simulink model "TEST_simulink"  (R2022b)
settings: Solver=VariableStepAuto  StartTime=0.0  StopTime=10.0  RelTol=1e-3
undefined symbols (not defined in the file): c0, c1, GFl_Final_vlaue, GFl_Initial_value, GFl_P_primary, GFl_Q_set, GFl_Sample_time, GFl_Step_time, GFm_Final_vlaue, GFm_Initial_value, GFm_P_primary, GFm_Q_set, GFm_Sample_time, GFm_Step_time, GFm_V_set_phph, GFmAIC_f_set, GFmAIC_Final_vlaue, GFmAIC_Initial_value, GFmAIC_P_primary, GFmAIC_P_set, GFmAIC_Q_set, GFmAIC_Sample_time, GFmAIC_Step_time, l0, l1, r0, r1, SG_f_set, SG_Final_vlaue, SG_Initial_value, SG_P_primary, SG_Q_set, SG_Sample_time, SG_Step_time, SG_V_set_phph, sigbuilder_block, V1_L1, V1_Ph_Ph, V1_R1, V2_L1, V2_Ph_Ph, V2_R1
libraries: Model_DG_Grid_Forming_Converter x30, Model_DG_Grid_Following_Converter x15, simulink x15, Model_DG_Synchronous_Generator x15, spsThreePhaseVIMeasurementLib x14, spsThreePhasePISectionLineLib x14, spsThreePhaseBreakerLib x6, spsThreePhaseFaultLib x3, spsThreePhaseParallelRLCLoadLib x2, spsThreePhaseTransformerTwoWindingsLib x2, spspowerguiLib x1
(part 1 of 6)
settings Model: Creator=r.dong  LastModifiedBy=r.dong

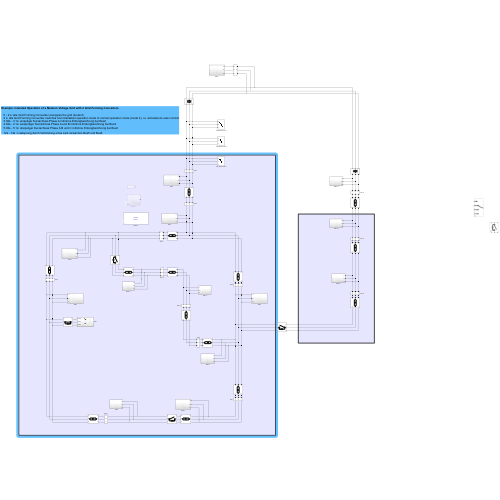
[thumbnail: Simulink's stored preview of the top-level diagram]
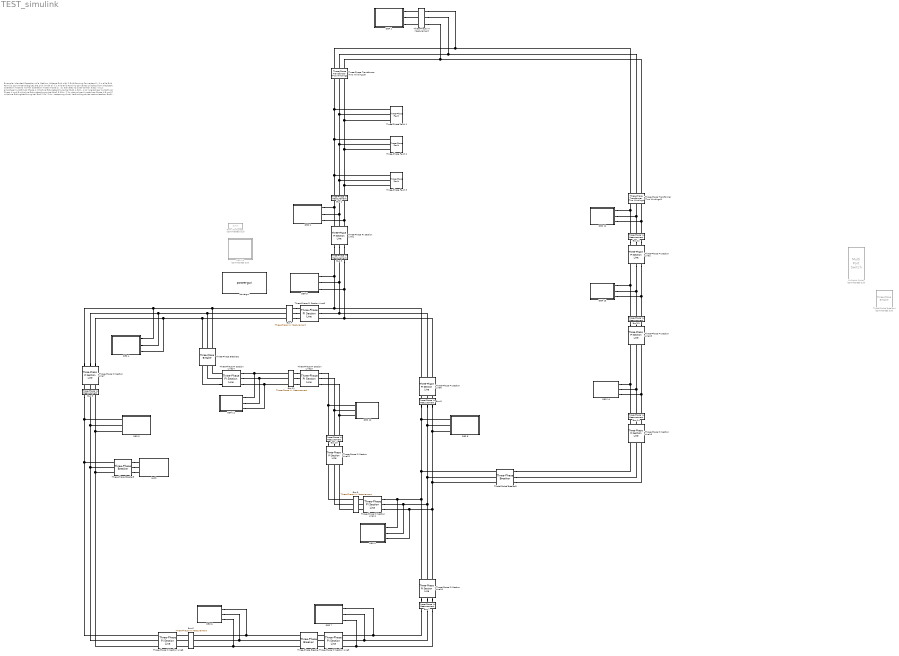
== system TEST_simulink ==
  note: Example: Islanded Operation of a Medium Voltage Grid with 2 Grid-Forming Converters
      |
      | 0 - 2 s: alle Grid Forming Conventer energizes the grid (mode 0)
      | 2 s: alle Grid Forming Conventer switches from blackstart operation mode to normal operation mode (mode 2), i.e. activates its outer control
      | 3.02s - 3.1s: einpoliger Kurzschluss Phase A mit/ohne Erdungberührung bei Bus2
      | 4.02s - 4.1s: zweipoliger Kurzschluss Phase A und B mit/ohne Erdungberührung bei Bus2
      | 5.02s - 5.1s: dreipoliger Kurzschluss Phase A B und C mit/ohne Erdungberührung bei Bus2
      |
      | 12s - 14s : Lastsprung durch Verbindung eines Last zwieschen Bus5 und Bus6
  Bus 10 : spsThreePhaseVIMeasurementLib/Three-Phase V-I Measurement  VoltageMeasurement=phase-to-phase  SetLabelV=on  LabelV=Vabc_10  Vpu=off  VpuLL=off  CurrentMeasurement=yes  SetLabelI=on  LabelI=Iabc_10  Ipu=off  Pbase=100e6  Vbase=500e3  OutputType=Complex  PhasorSimulation=off  PSBequivalent=0
  Bus 11 : spsThreePhaseVIMeasurementLib/Three-Phase V-I Measurement  VoltageMeasurement=phase-to-phase  SetLabelV=on  LabelV=Vabc_11  Vpu=off  VpuLL=off  CurrentMeasurement=yes  SetLabelI=on  LabelI=Iabc_11  Ipu=off  Pbase=100e6  Vbase=500e3  OutputType=Complex  PhasorSimulation=off  PSBequivalent=0
  Bus 12 : spsThreePhaseVIMeasurementLib/Three-Phase V-I Measurement  VoltageMeasurement=phase-to-phase  SetLabelV=on  LabelV=Vabc_12  Vpu=off  VpuLL=off  CurrentMeasurement=yes  SetLabelI=on  LabelI=Iabc_12  Ipu=off  Pbase=100e6  Vbase=500e3  OutputType=Complex  PhasorSimulation=off  PSBequivalent=0
  Bus 13 : spsThreePhaseVIMeasurementLib/Three-Phase V-I Measurement  VoltageMeasurement=phase-to-phase  SetLabelV=on  LabelV=Vabc_13  Vpu=off  VpuLL=off  CurrentMeasurement=yes  SetLabelI=on  LabelI=Iabc_13  Ipu=off  Pbase=100e6  Vbase=500e3  OutputType=Complex  PhasorSimulation=off  PSBequivalent=0
  Bus 14 : spsThreePhaseVIMeasurementLib/Three-Phase V-I Measurement  VoltageMeasurement=phase-to-phase  SetLabelV=on  LabelV=Vabc_14  Vpu=off  VpuLL=off  CurrentMeasurement=yes  SetLabelI=on  LabelI=Iabc_14  Ipu=off  Pbase=100e6  Vbase=500e3  OutputType=Complex  PhasorSimulation=off  PSBequivalent=0
  Bus 2 : spsThreePhaseVIMeasurementLib/Three-Phase V-I Measurement  VoltageMeasurement=phase-to-phase  SetLabelV=on  LabelV=Vabc_1  Vpu=off  VpuLL=off  CurrentMeasurement=yes  SetLabelI=on  LabelI=Iabc_1  Ipu=off  Pbase=100e6  Vbase=500e3  OutputType=Complex  PhasorSimulation=off  PSBequivalent=0
  Bus 3 : spsThreePhaseVIMeasurementLib/Three-Phase V-I Measurement  VoltageMeasurement=phase-to-ground  SetLabelV=on  LabelV=Vabc_3  Vpu=off  VpuLL=off  CurrentMeasurement=yes  SetLabelI=on  LabelI=Iabc_3  Ipu=off  Pbase=100e6  Vbase=500e3  OutputType=Complex  PhasorSimulation=off  PSBequivalent=0
  Bus 4 : spsThreePhaseVIMeasurementLib/Three-Phase V-I Measurement  VoltageMeasurement=phase-to-phase  SetLabelV=on  LabelV=Vabc_4  Vpu=off  VpuLL=off  CurrentMeasurement=yes  SetLabelI=on  LabelI=Iabc_4  Ipu=off  Pbase=100e6  Vbase=500e3  OutputType=Complex  PhasorSimulation=off  PSBequivalent=0
  Bus 5 : spsThreePhaseVIMeasurementLib/Three-Phase V-I Measurement  VoltageMeasurement=phase-to-phase  SetLabelV=on  LabelV=Vabc_5  Vpu=off  VpuLL=off  CurrentMeasurement=yes  SetLabelI=on  LabelI=Iabc_5  Ipu=off  Pbase=100e6  Vbase=500e3  OutputType=Complex  PhasorSimulation=off  PSBequivalent=0
  Bus 6 : spsThreePhaseVIMeasurementLib/Three-Phase V-I Measurement  VoltageMeasurement=phase-to-phase  SetLabelV=on  LabelV=Vabc_6  Vpu=off  VpuLL=off  CurrentMeasurement=yes  SetLabelI=on  LabelI=Iabc_6  Ipu=off  Pbase=100e6  Vbase=500e3  OutputType=Complex  PhasorSimulation=off  PSBequivalent=0
  Bus 7 : spsThreePhaseVIMeasurementLib/Three-Phase V-I Measurement  VoltageMeasurement=phase-to-phase  SetLabelV=on  LabelV=Vabc_7  Vpu=off  VpuLL=off  CurrentMeasurement=yes  SetLabelI=on  LabelI=Iabc_7  Ipu=off  Pbase=100e6  Vbase=500e3  OutputType=Complex  PhasorSimulation=off  PSBequivalent=0
  Bus 8 : spsThreePhaseVIMeasurementLib/Three-Phase V-I Measurement  VoltageMeasurement=phase-to-phase  SetLabelV=on  LabelV=Vabc_8  Vpu=off  VpuLL=off  CurrentMeasurement=yes  SetLabelI=on  LabelI=Iabc_8  Ipu=off  Pbase=100e6  Vbase=500e3  OutputType=Complex  PhasorSimulation=off  PSBequivalent=0
  Bus 9 : spsThreePhaseVIMeasurementLib/Three-Phase V-I Measurement  VoltageMeasurement=phase-to-phase  SetLabelV=on  LabelV=Vabc_9  Vpu=off  VpuLL=off  CurrentMeasurement=yes  SetLabelI=on  LabelI=Iabc_9  Ipu=off  Pbase=100e6  Vbase=500e3  OutputType=Complex  PhasorSimulation=off  PSBequivalent=0
  DER 1 : Subsystem
  DER 10 : Subsystem
  DER 11 : Subsystem
  DER 12 : Subsystem
  DER 13 : Subsystem
  DER 14 : Subsystem
  DER 15 : Subsystem  Commented=on
  DER 2 : Subsystem
  DER 3 : Subsystem
  DER 4 : Subsystem
  DER 5 : Subsystem
  DER 6 : Subsystem
  DER 7 : Subsystem
  DER 8 : Subsystem
  DER 9 : Subsystem
  From Workspace : FromWorkspace  Commented=on  VariableName=simin
  Last1 : Subsystem
  Multiport Switch : MultiPortSwitch  Commented=on  SaturateOnIntegerOverflow=off  InputSameDT=off
  Three-Phase PI Section Line1 : spsThreePhasePISectionLineLib/Three-Phase PI Section Line  LConnTagsString=a|b|c  RConnTagsString=A|B|C  Length=2.8  Frequency=50  Resistances=[ r1 r0]  Inductances="[ l1  l0]"  Capacitances=[c1 c0]
  Three-Phase PI Section Line10 : spsThreePhasePISectionLineLib/Three-Phase PI Section Line  LConnTagsString=a|b|c  RConnTagsString=A|B|C  Length=1.7  Frequency=50  Resistances=[ r1 r0]  Inductances="[ l1  l0]"  Capacitances=[c1 c0]
  Three-Phase PI Section Line11 : spsThreePhasePISectionLineLib/Three-Phase PI Section Line  LConnTagsString=a|b|c  RConnTagsString=A|B|C  Length=4.4  Frequency=50  Resistances=[ r1 r0]  Inductances="[ l1  l0]"  Capacitances=[c1 c0]
  Three-Phase PI Section Line12 : spsThreePhasePISectionLineLib/Three-Phase PI Section Line  LConnTagsString=a|b|c  RConnTagsString=A|B|C  Length=0.8  Frequency=50  Resistances=[ r1 r0]  Inductances="[ l1  l0]"  Capacitances=[c1 c0]
  Three-Phase PI Section Line13 : spsThreePhasePISectionLineLib/Three-Phase PI Section Line  LConnTagsString=a|b|c  RConnTagsString=A|B|C  Length=0.3  Frequency=50  Resistances=[ r1 r0]  Inductances="[ l1  l0]"  Capacitances=[c1 c0]
  Three-Phase PI Section Line14 : spsThreePhasePISectionLineLib/Three-Phase PI Section Line  LConnTagsString=a|b|c  RConnTagsString=A|B|C  Length=4.4  Frequency=50  Resistances=[ r1 r0]  Inductances="[ l1  l0]"  Capacitances=[c1 c0]
  Three-Phase PI Section Line15 : spsThreePhasePISectionLineLib/Three-Phase PI Section Line  LConnTagsString=a|b|c  RConnTagsString=A|B|C  Length=3  Frequency=50  Resistances=[ r1 r0]  Inductances="[ l1  l0]"  Capacitances=[c1 c0]
  Three-Phase PI Section Line16 : spsThreePhasePISectionLineLib/Three-Phase PI Section Line  LConnTagsString=a|b|c  RConnTagsString=A|B|C  Length=2  Frequency=50  Resistances=[ r1 r0]  Inductances="[ l1  l0]"  Capacitances=[c1 c0]
  Three-Phase PI Section Line2 : spsThreePhasePISectionLineLib/Three-Phase PI Section Line  LConnTagsString=a|b|c  RConnTagsString=A|B|C  Length=4.9  Frequency=50  Resistances=[ r1 r0]  Inductances="[ l1  l0]"  Capacitances=[c1 c0]
  Three-Phase PI Section Line5 : spsThreePhasePISectionLineLib/Three-Phase PI Section Line  LConnTagsString=a|b|c  RConnTagsString=A|B|C  Length=0.6  Frequency=50  Resistances=[ r1 r0]  Inductances="[ l1  l0]"  Capacitances=[c1 c0]
  Three-Phase PI Section Line6 : spsThreePhasePISectionLineLib/Three-Phase PI Section Line  LConnTagsString=a|b|c  RConnTagsString=A|B|C  Length=4.4  Frequency=50  Resistances=[ r1 r0]  Inductances="[ l1  l0]"  Capacitances=[c1 c0]
  Three-Phase PI Section Line7 : spsThreePhasePISectionLineLib/Three-Phase PI Section Line  LConnTagsString=a|b|c  RConnTagsString=A|B|C  Length=0.6  Frequency=50  Resistances=[ r1 r0]  Inductances="[ l1  l0]"  Capacitances=[c1 c0]
  Three-Phase PI Section Line8 : spsThreePhasePISectionLineLib/Three-Phase PI Section Line  LConnTagsString=a|b|c  RConnTagsString=A|B|C  Length=1.5  Frequency=50  Resistances=[ r1 r0]  Inductances="[ l1  l0]"  Capacitances=[c1 c0]
  Three-Phase PI Section Line9 : spsThreePhasePISectionLineLib/Three-Phase PI Section Line  LConnTagsString=a|b|c  RConnTagsString=A|B|C  Length=0.2  Frequency=50  Resistances=[ r1 r0]  Inductances="[ l1  l0]"  Capacitances=[c1 c0]
  Three-Phase Transformer (Two Windings)1 : spsThreePhaseTransformerTwoWindingsLib/Three-Phase Transformer (Two Windings)  Winding1Connection=Yg  Winding2Connection=Yg  CoreType=Three single-phase transformers  SetSaturation=off  Hysteresis=off  DataFile='hysteresis'  SetInitialFlux=off  Measurements=None  UNITS=pu  NominalPower=[ 1 , 50 ]  Winding1=[V1_Ph_Ph,V1_R1,V1_L1 ]  Winding2=[V2_Ph_Ph,V2_R1,V2_L1 ]  Rm=Rm  Lm=Lm  L0=0.5  Saturation=[ 0,0 ; 0.0024,1.2 ; 1.0,1.52 ]  InitialFluxes=[ 0.8 , -0.8 , 0.7 ]  BreakLoop=off  DiscreteSolver=Trapezoidal iterative  DataType=off  TransfoNumber=1
  Three-Phase Transformer (Two Windings)3 : spsThreePhaseTransformerTwoWindingsLib/Three-Phase Transformer (Two Windings)  Winding1Connection=Yg  Winding2Connection=Yg  CoreType=Three single-phase transformers  SetSaturation=off  Hysteresis=off  DataFile='hysteresis'  SetInitialFlux=off  Measurements=None  UNITS=pu  NominalPower=[ 1 , 50 ]  Winding1=[V1_Ph_Ph,V1_R1,V1_L1 ]  Winding2=[V2_Ph_Ph,V2_R1,V2_L1 ]  Rm=Rm  Lm=Lm  L0=0.5  Saturation=[ 0,0 ; 0.0024,1.2 ; 1.0,1.52 ]  InitialFluxes=[ 0.8 , -0.8 , 0.7 ]  BreakLoop=off  DiscreteSolver=Trapezoidal iterative  DataType=off  TransfoNumber=1
  Three-Phase V-I Measurement : spsThreePhaseVIMeasurementLib/Three-Phase V-I Measurement  VoltageMeasurement=no  SetLabelV=off  LabelV=Vabc  Vpu=off  VpuLL=off  CurrentMeasurement=no  SetLabelI=off  LabelI=Iabc  Ipu=off  Pbase=100e6  Vbase=500e3  OutputType=Complex  PhasorSimulation=off  PSBequivalent=0
  Three-Phase Breaker1 : spsThreePhaseBreakerLib/Three-Phase Breaker  InitialState=open  SwitchA=on  SwitchB=on  SwitchC=on  SwitchTimes=Break1_switching_time  External=off  BreakerResistance=Break1_Ron  SnubberResistance=Break1_Rs  SnubberCapacitance=Break1_Cs  Measurements=None
  Three-Phase Breaker2 : spsThreePhaseBreakerLib/Three-Phase Breaker  InitialState=open  SwitchA=on  SwitchB=on  SwitchC=on  SwitchTimes=Break2_switching_time  External=off  BreakerResistance=Break2_Ron  SnubberResistance=Break2_Rs  SnubberCapacitance=Break2_Cs  Measurements=None
  Three-Phase Breaker3 : spsThreePhaseBreakerLib/Three-Phase Breaker  InitialState=open  SwitchA=on  SwitchB=on  SwitchC=on  SwitchTimes=Break3_switching_time  External=off  BreakerResistance=Break3_Ron  SnubberResistance=Break3_Rs  SnubberCapacitance=Break3_Cs  Measurements=None
  Three-Phase Breaker4 : spsThreePhaseBreakerLib/Three-Phase Breaker  Commented=on  InitialState=open  SwitchA=on  SwitchB=on  SwitchC=on  SwitchTimes=Break2_switching_time  External=off  BreakerResistance=Break2_Ron  SnubberResistance=Break2_Rs  SnubberCapacitance=Break2_Cs  Measurements=None
  Three-Phase Breaker5 : spsThreePhaseBreakerLib/Three-Phase Breaker  InitialState=closed  SwitchA=on  SwitchB=on  SwitchC=on  SwitchTimes=14  External=off  BreakerResistance=Break2_Ron  SnubberResistance=Break2_Rs  SnubberCapacitance=Break2_Cs  Measurements=None
  Three-Phase Fault 1 : spsThreePhaseFaultLib/Three-Phase Fault  InitialStates=0  FaultA=on  FaultB=off  FaultC=off  GroundFault=off  SwitchTimes=Fault1_Break_switching_time  External=off  SwitchStatus=NaN  FaultResistance=Fault1_Ron  GroundResistance=Fault1_Rg  SnubberResistance=Fault1_Rs  SnubberCapacitance=Fault1_Cs  Measurements=None
  Three-Phase Fault 2 : spsThreePhaseFaultLib/Three-Phase Fault  InitialStates=0  FaultA=on  FaultB=on  FaultC=off  GroundFault=off  SwitchTimes=Fault2_Break_switching_time  External=off  SwitchStatus=NaN  FaultResistance=Fault2_Ron  GroundResistance=Fault2_Rg  SnubberResistance=Fault2_Rs  SnubberCapacitance=Fault2_Cs  Measurements=None
  Three-Phase Fault 3 : spsThreePhaseFaultLib/Three-Phase Fault  InitialStates=0  FaultA=on  FaultB=on  FaultC=on  GroundFault=off  SwitchTimes=Fault3_Break_switching_time  External=off  SwitchStatus=NaN  FaultResistance=Fault3_Ron  GroundResistance=Fault3_Rg  SnubberResistance=Fault3_Rs  SnubberCapacitance=Fault3_Cs  Measurements=None
  powergui : spspowerguiLib/powergui  Priority=1  SimulationMode=Discrete  SampleTime=1e-4  frequency=60  Iterations=50  frequencyindice=0  Pbase=100e6  ErrMax=1e-4  UnitsV=kV  UnitsW=MW  buscounter=0  FunctionMessages=off  echomessages=off  EnableUseOfTLC=off  CurrentSourceSwitches=off  DisableSnubberDevices=off  DisableRonSwitches=off  DisableVfSwitches=off  DisplayEquations=off  AutomaticDiscreteSolvers=off  SolverType=Backward Euler  Interpol=off  ExternalGateDelay=off  methode=off  Ts=100  x0status=blocks  SPID=on  SwTol=0  HookPort=off  NonlinearTolerance=1e-4  nMaxIteration=100  ContinueOnMaxIteration=off  RestoreLinks=warning  ResistiveCurrentMeasurement=off  Frange=[0:2:500]  Ylog=off  Xlog=on  ShowGrid=off  save=off  variable=ZData  structure=0  ZoomFFT=off  StartTime=0.0  cycles=1  DisplayStyle=1  fundamental=60  FreqAxis=off  MaxFrequency=1000  frequencyindicesteady=1  RmsSteady=1  display=off
  connections:
  Three-Phase PI Section Line5/LConn1 -- Three-Phase PI Section Line6/LConn1 -- DER 3/RConn1 -- Bus 3/RConn1
  Bus 12/LConn2 -- DER 12/RConn2 -- Three-Phase Transformer (Two Windings)1/RConn2
  Three-Phase Breaker3/LConn1 -- Three-Phase PI Section Line16/RConn1
  Three-Phase Breaker1/LConn3 -- Bus 6/RConn3 -- DER 6/RConn3
  Three-Phase Breaker1/LConn1 -- Bus 6/RConn1 -- DER 6/RConn1
  Bus 12/LConn3 -- DER 12/RConn3 -- Three-Phase Transformer (Two Windings)1/RConn3
  Three-Phase PI Section Line13/LConn1 -- Bus 10/RConn1 -- DER 10/RConn1
  Three-Phase PI Section Line6/LConn2 -- Three-Phase PI Section Line5/LConn2 -- DER 3/RConn2 -- Bus 3/RConn2
  Three-Phase PI Section Line8/LConn3 -- Bus 5/RConn3 -- DER 5/RConn3 -- Three-Phase Breaker5/LConn3
  Bus 5/RConn2 -- DER 5/RConn2 -- Three-Phase Breaker5/LConn2 -- Three-Phase PI Section Line8/LConn2
  Bus 9/LConn3 -- Three-Phase PI Section Line12/LConn3
  Three-Phase PI Section Line2/RConn3 -- DER 13/RConn3 -- Bus 13/LConn3
  Three-Phase PI Section Line13/LConn3 -- DER 10/RConn3 -- Bus 10/RConn3
  Three-Phase PI Section Line14/LConn3 -- Bus 11/RConn3 -- DER 11/RConn3
  Three-Phase PI Section Line11/LConn2 -- Bus 8/LConn2 -- DER 8/RConn2 -- Three-Phase Breaker3/RConn2 -- Three-Phase PI Section Line10/RConn2 -- DER 9/RConn2
  Bus 5/RConn1 -- DER 5/RConn1 -- Three-Phase Breaker5/LConn1 -- Three-Phase PI Section Line8/LConn1
  Bus 9/LConn2 -- Three-Phase PI Section Line12/LConn2
  Three-Phase Transformer (Two Windings)1/LConn1 -- Three-Phase V-I Measurement/RConn1 -- Three-Phase Transformer (Two Windings)3/LConn1
  Three-Phase PI Section Line7/LConn1 -- Three-Phase Breaker2/LConn1 -- Bus 4/RConn1 -- DER 4/RConn1
  Three-Phase PI Section Line2/RConn2 -- DER 13/RConn2 -- Bus 13/LConn2
  Three-Phase PI Section Line11/LConn3 -- DER 8/RConn3 -- Bus 8/LConn3 -- Three-Phase Breaker3/RConn3 -- Three-Phase PI Section Line10/RConn3 -- DER 9/RConn3
  Bus 9/LConn1 -- Three-Phase PI Section Line12/LConn1
  Three-Phase Breaker3/LConn2 -- Three-Phase PI Section Line16/RConn2
  Three-Phase Breaker3/RConn1 -- Bus 8/LConn1 -- DER 8/RConn1 -- DER 9/RConn1 -- Three-Phase PI Section Line11/LConn1 -- Three-Phase PI Section Line10/RConn1
  Three-Phase PI Section Line13/LConn2 -- Bus 10/RConn2 -- DER 10/RConn2
  Three-Phase Breaker1/LConn2 -- Bus 6/RConn2 -- DER 6/RConn2
  Three-Phase Transformer (Two Windings)3/LConn2 -- Three-Phase V-I Measurement/RConn2 -- Three-Phase Transformer (Two Windings)1/LConn2
  Three-Phase Breaker2/LConn2 -- DER 4/RConn2 -- Three-Phase PI Section Line7/LConn2 -- Bus 4/RConn2
  Bus 7/LConn1 -- DER 7/RConn1 -- Three-Phase PI Section Line9/RConn1
  Bus 13/LConn1 -- DER 13/RConn1 -- Three-Phase PI Section Line2/RConn1
  Bus 7/LConn2 -- Three-Phase PI Section Line9/RConn2 -- DER 7/RConn2
  Three-Phase PI Section Line7/LConn3 -- Three-Phase Breaker2/LConn3 -- Bus 4/RConn3 -- DER 4/RConn3
  Three-Phase PI Section Line1/LConn3 -- DER 2/RConn3 -- Bus 2/RConn3
  Three-Phase PI Section Line5/LConn3 -- Three-Phase PI Section Line6/LConn3 -- DER 3/RConn3 -- Bus 3/RConn3
  Bus 12/LConn1 -- DER 12/RConn1 -- Three-Phase Transformer (Two Windings)1/RConn1
  Three-Phase PI Section Line1/LConn1 -- DER 2/RConn1 -- Bus 2/RConn1
  Three-Phase PI Section Line14/LConn2 -- DER 11/RConn2 -- Bus 11/RConn2
  Three-Phase Breaker3/LConn3 -- Three-Phase PI Section Line16/RConn3
  Bus 7/LConn3 -- Three-Phase PI Section Line9/RConn3 -- DER 7/RConn3
  Three-Phase Transformer (Two Windings)1/LConn3 -- Three-Phase V-I Measurement/RConn3 -- Three-Phase Transformer (Two Windings)3/LConn3
  Three-Phase PI Section Line1/LConn2 -- DER 2/RConn2 -- Bus 2/RConn2
  Bus 13/RConn2 -- Three-Phase PI Section Line15/LConn2
  Bus 4/LConn2 -- Three-Phase PI Section Line5/RConn2
  Bus 13/RConn3 -- Three-Phase PI Section Line15/LConn3
  Three-Phase PI Section Line10/LConn3 -- Bus 7/RConn3
  Bus 12/RConn1 -- Three-Phase PI Section Line2/LConn1
  Bus 12/RConn3 -- Three-Phase PI Section Line2/LConn3
  Bus 6/LConn2 -- Three-Phase PI Section Line8/RConn2
  Bus 5/LConn2 -- Three-Phase PI Section Line7/RConn2
  Bus 14/LConn2 -- DER 14/RConn2 -- Three-Phase PI Section Line15/RConn2
  Three-Phase Fault 1/LConn3 -- Three-Phase Transformer (Two Windings)3/RConn3 -- Three-Phase Fault 3/LConn3 -- Bus 2/LConn3 -- Three-Phase Fault 2/LConn3
  Three-Phase PI Section Line1/RConn3 -- Bus 3/LConn3
  Three-Phase Fault 1/LConn2 -- Three-Phase Transformer (Two Windings)3/RConn2 -- Three-Phase Fault 2/LConn2 -- Three-Phase Fault 3/LConn2 -- Bus 2/LConn2
  Bus 13/RConn1 -- Three-Phase PI Section Line15/LConn1
  Three-Phase PI Section Line16/LConn1 -- Bus 14/RConn1
  Bus 10/LConn2 -- Three-Phase PI Section Line12/RConn2
  Three-Phase PI Section Line11/RConn1 -- Bus 9/RConn1
  Three-Phase PI Section Line16/LConn3 -- Bus 14/RConn3
  Bus 4/LConn3 -- Three-Phase PI Section Line5/RConn3
  Bus 10/LConn1 -- Three-Phase PI Section Line12/RConn1
  Three-Phase Fault 1/LConn1 -- Three-Phase Transformer (Two Windings)3/RConn1 -- Three-Phase Fault 2/LConn1 -- Three-Phase Fault 3/LConn1 -- Bus 2/LConn1
  Bus 14/LConn1 -- DER 14/RConn1 -- Three-Phase PI Section Line15/RConn1
  Bus 5/LConn3 -- Three-Phase PI Section Line7/RConn3
  Bus 10/LConn3 -- Three-Phase PI Section Line12/RConn3
  Bus 11/LConn3 -- Three-Phase PI Section Line13/RConn3
  Three-Phase PI Section Line11/RConn2 -- Bus 9/RConn2
  Three-Phase PI Section Line14/RConn1 -- Three-Phase Breaker2/RConn1
  Three-Phase PI Section Line16/LConn2 -- Bus 14/RConn2
  Bus 6/LConn3 -- Three-Phase PI Section Line8/RConn3
  Three-Phase PI Section Line6/RConn3 -- Bus 8/RConn3
  Three-Phase PI Section Line6/RConn2 -- Bus 8/RConn2
  Three-Phase PI Section Line14/RConn2 -- Three-Phase Breaker2/RConn2
  Three-Phase PI Section Line9/LConn1 -- Three-Phase Breaker1/RConn1
  Bus 11/LConn2 -- Three-Phase PI Section Line13/RConn2
  Three-Phase PI Section Line10/LConn1 -- Bus 7/RConn1
  Three-Phase PI Section Line14/RConn3 -- Three-Phase Breaker2/RConn3
  Three-Phase PI Section Line1/RConn1 -- Bus 3/LConn1
  Bus 6/LConn1 -- Three-Phase PI Section Line8/RConn1
  Three-Phase PI Section Line6/RConn1 -- Bus 8/RConn1
  Three-Phase PI Section Line11/RConn3 -- Bus 9/RConn3
  Bus 11/LConn1 -- Three-Phase PI Section Line13/RConn1
  Three-Phase PI Section Line9/LConn3 -- Three-Phase Breaker1/RConn3
  Three-Phase PI Section Line10/LConn2 -- Bus 7/RConn2
  Three-Phase PI Section Line9/LConn2 -- Three-Phase Breaker1/RConn2
  Bus 4/LConn1 -- Three-Phase PI Section Line5/RConn1
  Bus 12/RConn2 -- Three-Phase PI Section Line2/LConn2
  Three-Phase PI Section Line1/RConn2 -- Bus 3/LConn2
  Bus 5/LConn1 -- Three-Phase PI Section Line7/RConn1
  Bus 14/LConn3 -- DER 14/RConn3 -- Three-Phase PI Section Line15/RConn3
  Three-Phase PI Section Line14/LConn1 -- DER 11/RConn1 -- Bus 11/RConn1
  DER 1/RConn1 -- Three-Phase V-I Measurement/LConn1
  DER 1/RConn2 -- Three-Phase V-I Measurement/LConn2
  DER 1/RConn3 -- Three-Phase V-I Measurement/LConn3
  Three-Phase Breaker5/RConn1 -- Last1/LConn1
  Three-Phase Breaker5/RConn2 -- Last1/LConn2
  Three-Phase Breaker5/RConn3 -- Last1/LConn3

== system TEST_simulink/DER 1 ==
  Grid Following Conventer : Subsystem  Commented=on
  Grid Forming Conventer : Subsystem  Commented=on
  Grid Forming Converter AIC : Subsystem  Commented=on
  SG : Subsystem
  L1 : PMIOPort  Side=Right
  L2 : PMIOPort  Port=2  Side=Right
  L3 : PMIOPort  Port=3  Side=Right
  connections:
  SG/RConn1 -- Grid Forming Converter AIC/RConn1 -- L1/RConn1 -- Grid Forming Converter AIC/RConn3 -- Grid Forming Converter AIC/RConn2 -- Grid Forming Conventer/RConn1 -- Grid Following Conventer/RConn1
  SG/RConn2 -- L2/RConn1 -- Grid Forming Conventer/RConn2 -- Grid Following Conventer/RConn2
  SG/RConn3 -- L3/RConn1 -- Grid Forming Conventer/RConn3 -- Grid Following Conventer/RConn3

== system TEST_simulink/DER 10 ==
  Grid Following Conventer : Subsystem  Commented=on
  Grid Forming Conventer : Subsystem  Commented=on
  Grid Forming Converter AIC : Subsystem  Commented=on
  SG : Subsystem  Commented=on
  L1 : PMIOPort  Side=Right
  L2 : PMIOPort  Port=2  Side=Right
  L3 : PMIOPort  Port=3  Side=Right
  connections:
  L3/RConn1 -- SG/RConn3 -- Grid Following Conventer/RConn3 -- Grid Forming Conventer/RConn3
  L2/RConn1 -- SG/RConn2 -- Grid Following Conventer/RConn2 -- Grid Forming Conventer/RConn2
  L1/RConn1 -- Grid Forming Converter AIC/RConn1 -- SG/RConn1 -- Grid Following Conventer/RConn1 -- Grid Forming Conventer/RConn1 -- Grid Forming Converter AIC/RConn2 -- Grid Forming Converter AIC/RConn3

== system TEST_simulink/DER 11 ==
  Grid Following Conventer : Subsystem  Commented=on
  Grid Forming Conventer : Subsystem  Commented=on
  Grid Forming Converter AIC : Subsystem  Commented=on
  SG : Subsystem  Commented=on
  L1 : PMIOPort  Side=Right
  L2 : PMIOPort  Port=2  Side=Right
  L3 : PMIOPort  Port=3  Side=Right
  connections:
  Grid Forming Converter AIC/RConn3 -- Grid Forming Converter AIC/RConn2 -- Grid Forming Conventer/RConn1 -- Grid Following Conventer/RConn1 -- SG/RConn1 -- Grid Forming Converter AIC/RConn1 -- L1/RConn1
  Grid Forming Conventer/RConn2 -- Grid Following Conventer/RConn2 -- SG/RConn2 -- L2/RConn1
  Grid Forming Conventer/RConn3 -- Grid Following Conventer/RConn3 -- SG/RConn3 -- L3/RConn1

== system TEST_simulink/DER 12 ==
  Grid Following Conventer : Subsystem  Commented=on
  Grid Forming Conventer : Subsystem  Commented=on
  Grid Forming Converter AIC : Subsystem  Commented=on
  SG : Subsystem  Commented=on
  L1 : PMIOPort  Side=Right
  L2 : PMIOPort  Port=2  Side=Right
  L3 : PMIOPort  Port=3  Side=Right
  connections:
  Grid Forming Converter AIC/RConn3 -- Grid Forming Converter AIC/RConn2 -- Grid Forming Conventer/RConn1 -- Grid Following Conventer/RConn1 -- SG/RConn1 -- Grid Forming Converter AIC/RConn1 -- L1/RConn1
  Grid Forming Conventer/RConn2 -- Grid Following Conventer/RConn2 -- SG/RConn2 -- L2/RConn1
  Grid Forming Conventer/RConn3 -- Grid Following Conventer/RConn3 -- SG/RConn3 -- L3/RConn1

== system TEST_simulink/DER 13 ==
  Grid Following Conventer : Subsystem  Commented=on
  Grid Forming Conventer : Subsystem  Commented=on
  Grid Forming Converter AIC : Subsystem  Commented=on
  SG : Subsystem  Commented=on
  L1 : PMIOPort  Side=Right
  L2 : PMIOPort  Port=2  Side=Right
  L3 : PMIOPort  Port=3  Side=Right
  connections:
  Grid Forming Converter AIC/RConn3 -- Grid Forming Converter AIC/RConn2 -- Grid Forming Conventer/RConn1 -- Grid Following Conventer/RConn1 -- SG/RConn1 -- Grid Forming Converter AIC/RConn1 -- L1/RConn1
  Grid Forming Conventer/RConn2 -- Grid Following Conventer/RConn2 -- SG/RConn2 -- L2/RConn1
  Grid Forming Conventer/RConn3 -- Grid Following Conventer/RConn3 -- SG/RConn3 -- L3/RConn1

== system TEST_simulink/DER 14 ==
  Grid Following Conventer : Subsystem  Commented=on
  Grid Forming Conventer : Subsystem  Commented=on
  Grid Forming Converter AIC : Subsystem  Commented=on
  SG : Subsystem  Commented=on
  L1 : PMIOPort  Side=Right
  L2 : PMIOPort  Port=2  Side=Right
  L3 : PMIOPort  Port=3  Side=Right
  connections:
  Grid Forming Converter AIC/RConn3 -- Grid Forming Converter AIC/RConn2 -- Grid Forming Conventer/RConn1 -- Grid Following Conventer/RConn1 -- SG/RConn1 -- Grid Forming Converter AIC/RConn1 -- L1/RConn1
  Grid Forming Conventer/RConn2 -- Grid Following Conventer/RConn2 -- SG/RConn2 -- L2/RConn1
  Grid Forming Conventer/RConn3 -- Grid Following Conventer/RConn3 -- SG/RConn3 -- L3/RConn1

== system TEST_simulink/DER 15 ==
  Grid Following Conventer : Subsystem  Commented=on
  Grid Forming Conventer : Subsystem  Commented=on
  Grid Forming Converter AIC : Subsystem  Commented=on
  SG : Subsystem  Commented=on
  L1 : PMIOPort  Side=Right
  L2 : PMIOPort  Port=2  Side=Right
  L3 : PMIOPort  Port=3  Side=Right
  connections:
  L3/RConn1 -- SG/RConn3 -- Grid Following Conventer/RConn3 -- Grid Forming Conventer/RConn3
  L2/RConn1 -- SG/RConn2 -- Grid Following Conventer/RConn2 -- Grid Forming Conventer/RConn2
  L1/RConn1 -- Grid Forming Converter AIC/RConn1 -- SG/RConn1 -- Grid Following Conventer/RConn1 -- Grid Forming Conventer/RConn1 -- Grid Forming Converter AIC/RConn2 -- Grid Forming Converter AIC/RConn3

== system TEST_simulink/DER 2 ==
  Grid Following Conventer : Subsystem  Commented=on
  Grid Forming Conventer : Subsystem  Commented=on
  Grid Forming Converter AIC : Subsystem  Commented=on
  SG : Subsystem  Commented=on
  L1 : PMIOPort  Side=Right
  L2 : PMIOPort  Port=2  Side=Right
  L3 : PMIOPort  Port=3  Side=Right
  connections:
  L3/RConn1 -- SG/RConn3 -- Grid Following Conventer/RConn3 -- Grid Forming Conventer/RConn3
  L2/RConn1 -- SG/RConn2 -- Grid Following Conventer/RConn2 -- Grid Forming Conventer/RConn2
  L1/RConn1 -- Grid Forming Converter AIC/RConn1 -- SG/RConn1 -- Grid Following Conventer/RConn1 -- Grid Forming Conventer/RConn1 -- Grid Forming Converter AIC/RConn2 -- Grid Forming Converter AIC/RConn3

== system TEST_simulink/DER 3 ==
  Grid Following Conventer : Subsystem  Commented=on
  Grid Forming Conventer : Subsystem  Commented=on
  Grid Forming Converter AIC : Subsystem  Commented=on
  SG : Subsystem  Commented=on
  L1 : PMIOPort  Side=Right
  L2 : PMIOPort  Port=2  Side=Right
  L3 : PMIOPort  Port=3  Side=Right
  connections:
  Grid Forming Converter AIC/RConn2 -- Grid Forming Converter AIC/RConn1 -- Grid Forming Conventer/RConn1 -- Grid Following Conventer/RConn1 -- SG/RConn1 -- Grid Forming Converter AIC/RConn3 -- L1/RConn1
  Grid Following Conventer/RConn2 -- SG/RConn2 -- Grid Forming Conventer/RConn2 -- L2/RConn1
  Grid Following Conventer/RConn3 -- SG/RConn3 -- Grid Forming Conventer/RConn3 -- L3/RConn1

== system TEST_simulink/DER 4 ==
  Grid Following Conventer : Subsystem  Commented=on
  Grid Forming Conventer : Subsystem  Commented=on
  Grid Forming Converter AIC : Subsystem  Commented=on
  SG : Subsystem  Commented=on
  L1 : PMIOPort  Side=Right
  L2 : PMIOPort  Port=2  Side=Right
  L3 : PMIOPort  Port=3  Side=Right
  connections:
  L3/RConn1 -- Grid Forming Conventer/RConn3 -- SG/RConn3 -- Grid Following Conventer/RConn3
  L2/RConn1 -- Grid Forming Conventer/RConn2 -- SG/RConn2 -- Grid Following Conventer/RConn2
  L1/RConn1 -- Grid Forming Converter AIC/RConn3 -- Grid Forming Converter AIC/RConn2 -- Grid Forming Converter AIC/RConn1 -- Grid Forming Conventer/RConn1 -- SG/RConn1 -- Grid Following Conventer/RConn1

== system TEST_simulink/DER 5 ==
  Grid Following Conventer : Subsystem  Commented=on
  Grid Forming Conventer : Subsystem  Commented=on
  Grid Forming Converter AIC : Subsystem  Commented=on
  SG : Subsystem  Commented=on
  L1 : PMIOPort  Side=Right
  L2 : PMIOPort  Port=2  Side=Right
  L3 : PMIOPort  Port=3  Side=Right
  connections:
  L3/RConn1 -- Grid Forming Conventer/RConn3 -- SG/RConn3 -- Grid Following Conventer/RConn3
  Grid Following Conventer/RConn2 -- SG/RConn2 -- Grid Forming Conventer/RConn2 -- L2/RConn1
  L1/RConn1 -- Grid Forming Converter AIC/RConn3 -- Grid Forming Converter AIC/RConn2 -- Grid Forming Converter AIC/RConn1 -- Grid Forming Conventer/RConn1 -- SG/RConn1 -- Grid Following Conventer/RConn1

== system TEST_simulink/DER 6 ==
  Grid Following Conventer : Subsystem  Commented=on
  Grid Forming Conventer : Subsystem  Commented=on
  Grid Forming Converter AIC : Subsystem  Commented=on
  SG : Subsystem  Commented=on
  L1 : PMIOPort  Side=Right
  L2 : PMIOPort  Port=2  Side=Right
  L3 : PMIOPort  Port=3  Side=Right
  connections:
  Grid Forming Converter AIC/RConn3 -- Grid Forming Converter AIC/RConn2 -- Grid Forming Conventer/RConn1 -- Grid Following Conventer/RConn1 -- SG/RConn1 -- Grid Forming Converter AIC/RConn1 -- L1/RConn1
  Grid Forming Conventer/RConn2 -- Grid Following Conventer/RConn2 -- SG/RConn2 -- L2/RConn1
  Grid Forming Conventer/RConn3 -- Grid Following Conventer/RConn3 -- SG/RConn3 -- L3/RConn1

== system TEST_simulink/DER 7 ==
  Grid Following Conventer : Subsystem  Commented=on
  Grid Forming Conventer : Subsystem  Commented=on
  Grid Forming Converter AIC : Subsystem  Commented=on
  SG : Subsystem  Commented=on
  L1 : PMIOPort  Side=Right
  L2 : PMIOPort  Port=2  Side=Right
  L3 : PMIOPort  Port=3  Side=Right
  connections:
  L3/RConn1 -- SG/RConn3 -- Grid Following Conventer/RConn3 -- Grid Forming Conventer/RConn3
  L2/RConn1 -- SG/RConn2 -- Grid Following Conventer/RConn2 -- Grid Forming Conventer/RConn2
  L1/RConn1 -- Grid Forming Converter AIC/RConn1 -- SG/RConn1 -- Grid Following Conventer/RConn1 -- Grid Forming Conventer/RConn1 -- Grid Forming Converter AIC/RConn2 -- Grid Forming Converter AIC/RConn3

== system TEST_simulink/DER 8 ==
  Grid Following Conventer : Subsystem  Commented=on
  Grid Forming Conventer : Subsystem  Commented=on
  Grid Forming Converter AIC : Subsystem  Commented=on
  SG : Subsystem  Commented=on
  L1 : PMIOPort  Side=Right
  L2 : PMIOPort  Port=2  Side=Right
  L3 : PMIOPort  Port=3  Side=Right
  connections:
  L3/RConn1 -- SG/RConn3 -- Grid Following Conventer/RConn3 -- Grid Forming Conventer/RConn3
  L2/RConn1 -- SG/RConn2 -- Grid Following Conventer/RConn2 -- Grid Forming Conventer/RConn2
  L1/RConn1 -- Grid Forming Converter AIC/RConn1 -- SG/RConn1 -- Grid Following Conventer/RConn1 -- Grid Forming Conventer/RConn1 -- Grid Forming Converter AIC/RConn2 -- Grid Forming Converter AIC/RConn3

== system TEST_simulink/DER 9 ==
  Grid Following Conventer : Subsystem  Commented=on
  Grid Forming Conventer : Subsystem  Commented=on
  Grid Forming Converter AIC : Subsystem  Commented=on
  SG : Subsystem  Commented=on
  L1 : PMIOPort  Side=Right
  L2 : PMIOPort  Port=2  Side=Right
  L3 : PMIOPort  Port=3  Side=Right
  connections:
  Grid Forming Converter AIC/RConn3 -- Grid Forming Converter AIC/RConn2 -- Grid Forming Conventer/RConn1 -- Grid Following Conventer/RConn1 -- SG/RConn1 -- Grid Forming Converter AIC/RConn1 -- L1/RConn1
  Grid Forming Conventer/RConn2 -- Grid Following Conventer/RConn2 -- SG/RConn2 -- L2/RConn1
  Grid Forming Conventer/RConn3 -- Grid Following Conventer/RConn3 -- SG/RConn3 -- L3/RConn1

== system TEST_simulink/Last1 ==
  Three-Phase Parallel RLC Load1 : spsThreePhaseParallelRLCLoadLib/Three-Phase Parallel RLC Load  LConnTagsString=A|B|C  Configuration=Y (grounded)  NominalVoltage=Vrms  Vabc=[1e3 1e3 1e3]  Vabcp=[1e3 1e3 1e3]  NominalFrequency=50  UnbalancedPower=off  ActivePower=activePower  InductivePower=reactivePower  CapacitivePower=0  Pabc=[10e3 9e3 11e3]  QLabc=[100 90 110]  QCabc=[100 90 110]  Pabcp=[10e3 9e3 11e3]  QLabcp=[100 90 110]  QCabcp=[100 90 110]  Measurements=None  LoadType=constant Z
  Three-Phase Parallel RLC Load4 : spsThreePhaseParallelRLCLoadLib/Three-Phase Parallel RLC Load  LConnTagsString=A|B|C  Configuration=Y (grounded)  NominalVoltage=Vrms  Vabc=[1e3 1e3 1e3]  Vabcp=[1e3 1e3 1e3]  NominalFrequency=50  UnbalancedPower=off  ActivePower=activePower  InductivePower=reactivePower  CapacitivePower=0  Pabc=[10e3 9e3 11e3]  QLabc=[100 90 110]  QCabc=[100 90 110]  Pabcp=[10e3 9e3 11e3]  QLabcp=[100 90 110]  QCabcp=[100 90 110]  Measurements=None  LoadType=constant Z
  Three-Phase Breaker2 : spsThreePhaseBreakerLib/Three-Phase Breaker  InitialState=open  SwitchA=on  SwitchB=on  SwitchC=on  SwitchTimes=[12]  External=off  BreakerResistance=0.01  SnubberResistance=1e6  SnubberCapacitance=inf  Measurements=None
  Conn1 : PMIOPort  Side=Left
  Conn2 : PMIOPort  Port=2  Side=Left
  Conn3 : PMIOPort  Port=3  Side=Left
  connections:
  Three-Phase Parallel RLC Load4/LConn3 -- Three-Phase Breaker2/LConn3 -- Conn3/RConn1
  Three-Phase Parallel RLC Load4/LConn1 -- Conn1/RConn1 -- Three-Phase Breaker2/LConn1
  Three-Phase Parallel RLC Load4/LConn2 -- Conn2/RConn1 -- Three-Phase Breaker2/LConn2
  Three-Phase Breaker2/RConn1 -- Three-Phase Parallel RLC Load1/LConn1
  Three-Phase Breaker2/RConn2 -- Three-Phase Parallel RLC Load1/LConn2
  Three-Phase Breaker2/RConn3 -- Three-Phase Parallel RLC Load1/LConn3

== system TEST_simulink/DER 1/Grid Following Conventer ==
  Bus Selector1 : BusSelector  OutputSignals=controller.measurements.P_grid,controller.measurements.Q_grid,controller.PLL.f_PLL,physical.V_grid_abc
  Constant8 : Constant  Value=GFl_P_primary
  Constant9 : Constant  Value=GFl_Q_set
  Gain : Gain  Gain=50
  Grid-Following Converter (3-phase)1 : Model_DG_Grid_Following_Converter/Grid-Following Converter (3-phase)  S_n=2e6  P_binst=1.5e6  V_n_phph=690  f_n=50  send_messages=on  T_s_ctrl=1e-3  T_s_PWM_meas=1e-4  T_s_SPS=1e-4  datatype='double'  swModeling=Average Model  f_sw=5e3  L_filter_conv_pu=[ 0.005 0.23 ]  C_filter_pu=[ 0.005 0.01 ]  L_filter_grid_pu=[ 0.01 0.04 ]  withTransformer=Grid coupling using transformer  V_n_grid_phph=20e3  RL_Trafo_Conv=[ 0.005 0.02 ]  RL_Trafo_Grid=[ 0.005 0.02 ]  Rm=500  Lm=500  meas_LPF=on  meas_LPF_f_cutoff=2500  prot_variant=tDMSquared warnings only  prot_v_ac_max=1.4  prot_t_ac_max=0.1  prot_v_ac_maxmax=1.25  prot_t_ac_maxmax=0.1  prot_v_ac_min=0.8  prot_t_ac_min=3  prot_v_ac_minmin=0.45  prot_t_ac_minmin=0.3  prot_f_ac_max=51.5  prot_t_f_ac_max=0.1  prot_f_ac_maxmax=52.5  prot_t_f_ac_maxmax=10  prot_f_ac_min=47.5  prot_t_f_ac_min=0.1  prot_i_ac_max=1.3  unitCtrlMode=VDE 4110  VDE4110_Pf_DBlow=49.8  VDE4110_Pf_DBhigh=50.2  VDE4110_Pf_droop=5  VDE4110_Pf_dPdt_max=1  VDE4110_Pf_T_LPF=33e-3  VDE4110_Pf_isStorage=on  VDE4110_Q_Mode=(c) Constant Q with Q(V)-limitation  VDE4110_Q_T_PT1=3.33  VDE4110_uq0ref=1  VDE4110_qmax=0.33  VDE4110_umax=1.04  VDE4110_deadband=0  VDE4110_p_pu=[0.1, 0.5, 0.6, 0.9, 1.0]  VDE4110_q_pu=[0.0, 0.0, -0.05, -0.33, -0.33]  VDE4110_p1=[0.94, 0.33]  VDE4110_p2=[0.96, 0]  VDE4110_p3=[1.04, 0]  VDE4110_p4=[1.06, -0.33]  VDE4110_cosphi_ref=1  VDE4110_Q_direction=Inductive Q injection  InnerCtrl_PQ_Ctrl_Mode=Closed loop  InnerCtrl_Kp_PQ=1  InnerCtrl_Ki_PQ=5  InnerCtrl_Kp=0.3  InnerCtrl_Ki=2  InnerCtrl_v_conv_max=1.25  InnerCtrl_i_conv_max=1.1  InnerCtrl_AD_activated=on  InnerCtrl_AD_Rvirt=0.1
      settings: SourceProductName=tDMSquared
  P_set_3 : Subsystem  Tag=STV Subsys  LoadFcn=sigbuilder_block('load');  StartFcn=sigbuilder_block('start');  StopFcn=sigbuilder_block('stop');  ClipboardFcn=sigbuilder_block('clipboard');  mask(Sigbuilder block){tuvar=[0:10]}
      mask help: Simulink:masks:SigbuilderBlock_MD
      mask init:
      | if ~strcmp(get_param(bdroot(gcbh),'SimulationStatus'),'stopped') tuvar = sigbuilder_block('maskInit'); end
      settings: CopyFcn=sigbuilder_block('copy');  DeleteFcn=sigbuilder_block('delete');  ModelCloseFcn=sigbuilder_block('modelClose');  PreSaveFcn=sigbuilder_block('preSave');  PauseFcn=sigbuilder_block('pause');  ContinueFcn=sigbuilder_block('continue');  NameChangeFcn=sigbuilder_block('namechange');  OpenFcn=sigbuilder_block('open',[-809.4 12.6 550.8 361.2 ]);  CloseFcn=sigbuilder_block('close');
      mask Display: plot(0, 0, 100, 100,[2, 2, 32, 32, 2], [68, 8, 8, 68, 68],[32, 2], [38, 38], [32, 19, 2],[53, 60, 44], [32, 17, 17, 2],[16, 16, 31, 31]);txt = getActiveGroup(gcbh);text(2, 100, txt,'verticalAlignment', 'top');
  Scope{6,10,12..13} (4 alike) : Scope
  Step5 : Step  Time=GFl_Step_time  Before=GFl_Initial_value  After=GFl_Final_vlaue  SampleTime=GFl_Sample_time
  a : PMIOPort  Side=Right
  b : PMIOPort  Port=2  Side=Right
  c : PMIOPort  Port=3  Side=Right
  wires:
  Step5/1 -> Grid-Following Converter (3-phase)1/4
  Grid-Following Converter (3-phase)1/1 -> [conv_1]
  Gain/1 -> Scope12/1
  [conv_1] -> Bus Selector1/1
  Bus Selector1/4 -> Scope13/1  "<V_grid_abc>"
  Bus Selector1/1 -> Scope6/1  "<P_grid>"
  Bus Selector1/2 -> Scope10/1  "<Q_grid>"
  Constant8/1 -> Grid-Following Converter (3-phase)1/1
  Bus Selector1/3 -> Gain/1  "<f_PLL>"
  P_set_3/1(P_set_1) -> Grid-Following Converter (3-phase)1/2
  Constant9/1 -> Grid-Following Converter (3-phase)1/3
  connections:
  b/RConn1 -- Grid-Following Converter (3-phase)1/RConn2
  c/RConn1 -- Grid-Following Converter (3-phase)1/RConn3
  a/RConn1 -- Grid-Following Converter (3-phase)1/RConn1

== system TEST_simulink/DER 1/Grid Forming Conventer ==
  Bus Selector : BusSelector  OutputSignals=controller.measurements.P_grid,controller.measurements.Q_grid,controller.inner_control.f,physical.V_dc,physical.V_grid_abc
  Constant : Constant  Value=GFm_P_primary
  Constant10 : Constant  Value=GFm_Q_set
  Constant4 : Constant  Value=GFmAIC_f_set
  Constant6 : Constant  Value=GFm_V_set_phph
  Grid_Forming_Converter1 : Model_DG_Grid_Forming_Converter/Grid_Forming_Converter  S_n=2e6  V_n_phph=690  f_n=50  send_messages=on  T_s_ctrl=1e-4  T_s_PWM_meas=1e-4  T_s_SPS=1e-4  datatype='double'  swModeling=Average Model  f_sw=5e3  L_filter_conv_pu=[ 0.001 0.05097 ]  C_filter_pu=[ 0.06875 0.04569 ]  L_filter_grid_pu=[ 0.01 0.04 ]  C_dc_pu=0.75  withTransformer=Grid coupling using transformer  V_n_grid_phph=20e3  RL_Trafo_Conv=[ 0.005 0.02 ]  RL_Trafo_Grid=[ 0.005 0.02 ]  Rm=500  Lm=500  meas_lowpass=on  meas_f_cutoff_lowpass=2500  meas_f_cutoff_posseq=20  prot_variant=tDMSquared warnings only  v_dc_max=1.2  v_ac_max=1.4  t_ac_max=0.1  v_ac_maxmax=1.25  t_ac_maxmax=0.1  v_ac_min=0.8  t_ac_min=3  v_ac_minmin=0.45  t_ac_minmin=0.3  f_ac_max=51.5  t_f_ac_max=0.1  f_ac_maxmax=52.5  t_f_ac_maxmax=10  f_ac_min=47.5  t_f_ac_min=0.1  i_ac_max=1.3  outerCtrlStrategy=Droop  OuterCtrl_droop_kP=0.05  OuterCtrl_droop_kQ=0.1  OuterCtrl_droop_TQ=0.2  OuterCtrl_ZDroop_kf=0.05  OuterCtrl_ZDroop_kV=0.1  OuterCtrl_ZDroop_kR=0  OuterCtrl_ZDroop_kX=1  OuterCtrl_ZDroop_TV=0.2  OuterCtrl_VSM_H=0.1  OuterCtrl_VSM_Kd=40  OuterCtrl_VSM_K=20  OuterCtrl_VSM_kQ=0.1  OuterCtrl_VSM_TQ=0.2  OuterCtrl_Dual_Kp=0.01  OuterCtrl_Dual_Kd=1e-4  OuterCtrl_Dual_kQ=0.1  OuterCtrl_Dual_TQ=0.2  OuterCtrl_Lvirt=0  InnerCtrl_K_p_V_cap_controller=0.8  InnerCtrl_K_i_V_cap_controller=0.5  InnerCtrl_K_p_I_conv_controller=3.3  InnerCtrl_K_i_I_conv_controller=16.5  InnerCtrl_v_conv_max=1.3  InnerCtrl_i_conv_max=1  InnerCtrl_Cff_V_cap_ctrl=disabled  InnerCtrl_Cff_I_conv_ctrl=disabled  InnerCtrl_K_ff_I_grid=enabled  InnerCtrl_K_ff_V_cap=enabled  InnerCtrl_i_lim_type=dq coordinate system  InnerCtrl_active_damping=enabled  InnerCtrl_AD_R_virt_pu=0.2
      settings: SourceProductName=tDMSquared
  Ground : Ground
  P_set_1 : Subsystem  Tag=STV Subsys  LoadFcn=sigbuilder_block('load');  StartFcn=sigbuilder_block('start');  StopFcn=sigbuilder_block('stop');  ClipboardFcn=sigbuilder_block('clipboard');  mask(Sigbuilder block){tuvar=[0:10]}
      mask help: Simulink:masks:SigbuilderBlock_MD
      mask init:
      | if ~strcmp(get_param(bdroot(gcbh),'SimulationStatus'),'stopped') tuvar = sigbuilder_block('maskInit'); end
      settings: CopyFcn=sigbuilder_block('copy');  DeleteFcn=sigbuilder_block('delete');  ModelCloseFcn=sigbuilder_block('modelClose');  PreSaveFcn=sigbuilder_block('preSave');  PauseFcn=sigbuilder_block('pause');  ContinueFcn=sigbuilder_block('continue');  NameChangeFcn=sigbuilder_block('namechange');  OpenFcn=sigbuilder_block('open',[-809.4 12.6 550.8 361.2 ]);  CloseFcn=sigbuilder_block('close');
      mask Display: plot(0, 0, 100, 100,[2, 2, 32, 32, 2], [68, 8, 8, 68, 68],[32, 2], [38, 38], [32, 19, 2],[53, 60, 44], [32, 17, 17, 2],[16, 16, 31, 31]);txt = getActiveGroup(gcbh);text(2, 100, txt,'verticalAlignment', 'top');
  Scope{1..5} (5 alike) : Scope
  Step5 : Step  Time=GFm_Step_time  Before=GFm_Initial_value  After=GFm_Final_vlaue  SampleTime=GFm_Sample_time
  a : PMIOPort  Side=Right
  b : PMIOPort  Port=2  Side=Right
  c : PMIOPort  Port=3  Side=Right
  wires:
  Bus Selector/5 -> Scope5/1  "<V_grid_abc>"
  Bus Selector/2 -> Scope2/1  "<Q_grid>"
  Bus Selector/3 -> Scope3/1  "<f>"
  Bus Selector/1 -> Scope1/1  "<P_grid>"
  Bus Selector/4 -> Scope4/1  "<V_dc>"
  Grid_Forming_Converter1/1 -> [conv_1]
  [conv_1] -> Bus Selector/1
  Constant/1 -> Grid_Forming_Converter1/1
  P_set_1/1(P_set_1) -> Grid_Forming_Converter1/2
  Constant10/1 -> Grid_Forming_Converter1/3
  Constant4/1 -> Grid_Forming_Converter1/4
  Constant6/1 -> Grid_Forming_Converter1/5
  Ground/1 -> Grid_Forming_Converter1/6
  Step5/1 -> Grid_Forming_Converter1/7
  connections:
  a/RConn1 -- Grid_Forming_Converter1/RConn1
  b/RConn1 -- Grid_Forming_Converter1/RConn2
  c/RConn1 -- Grid_Forming_Converter1/RConn3

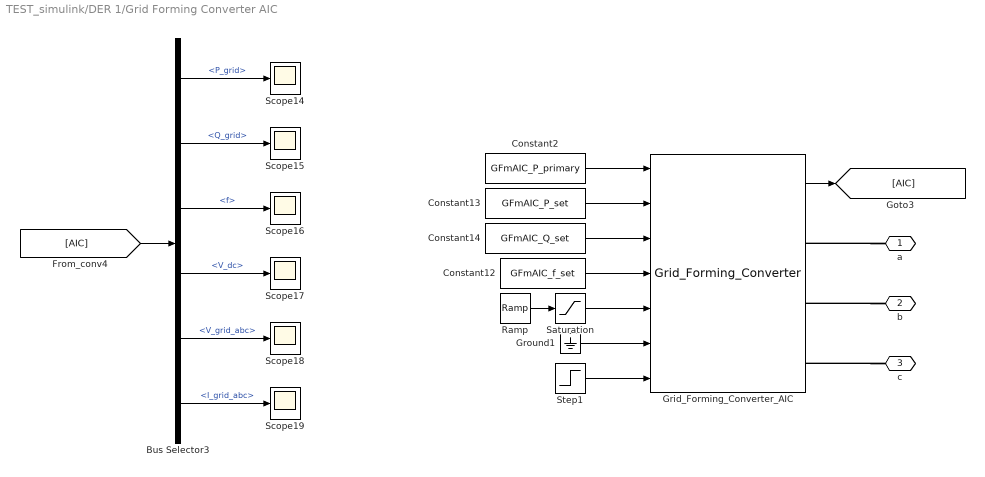
== system TEST_simulink/DER 1/Grid Forming Converter AIC ==
  Bus Selector3 : BusSelector  OutputSignals=controller.measurements.P_grid,controller.measurements.Q_grid,controller.inner_control.f,physical.V_dc,physical.V_grid_abc,physical.I_grid_abc
  Constant12 : Constant  Value=GFmAIC_f_set
  Constant13 : Constant  Value=GFmAIC_P_set
  Constant14 : Constant  Value=GFmAIC_Q_set
  Constant2 : Constant  Value=GFmAIC_P_primary
  Grid_Forming_Converter_AIC : Model_DG_Grid_Forming_Converter/Grid_Forming_Converter  S_n=100e3  V_n_phph=400  f_n=50  send_messages=on  T_s_ctrl=2e-4  T_s_PWM_meas=1e-5  T_s_SPS=1e-5  datatype='double'  swModeling=Average Model  f_sw=2.5e3  L_filter_conv_pu=[ 0.001 0.0177 ]  C_filter_pu=[ 0.000104 0.213 ]  L_filter_grid_pu=[ 0.001 0.00432 ]  C_dc_pu=0.75  withTransformer=Direct grid coupling of converter  V_n_grid_phph=400  RL_Trafo_Conv=[ 0.005 0.02 ]  RL_Trafo_Grid=[ 0.005 0.02 ]  Rm=500  Lm=500  meas_lowpass=on  meas_f_cutoff_lowpass=2500  meas_f_cutoff_posseq=20  prot_variant=tDMSquared warnings only  v_dc_max=1.2  v_ac_max=1.4  t_ac_max=0.1  v_ac_maxmax=1.25  t_ac_maxmax=0.1  v_ac_min=0.8  t_ac_min=3  v_ac_minmin=0.45  t_ac_minmin=0.3  f_ac_max=51.5  t_f_ac_max=0.1  f_ac_maxmax=52.5  t_f_ac_maxmax=10  f_ac_min=47.5  t_f_ac_min=0.1  i_ac_max=1.3  outerCtrlStrategy=Droop  OuterCtrl_droop_kP=0.05  OuterCtrl_droop_kQ=0.1  OuterCtrl_droop_TQ=0.2  OuterCtrl_ZDroop_kf=0.05  OuterCtrl_ZDroop_kV=0.1  OuterCtrl_ZDroop_kR=0  OuterCtrl_ZDroop_kX=1  OuterCtrl_ZDroop_TV=0.2  OuterCtrl_VSM_H=0.1  OuterCtrl_VSM_Kd=40  OuterCtrl_VSM_K=20  OuterCtrl_VSM_kQ=0.1  OuterCtrl_VSM_TQ=0.2  OuterCtrl_Dual_Kp=0.01  OuterCtrl_Dual_Kd=1e-4  OuterCtrl_Dual_kQ=0.1  OuterCtrl_Dual_TQ=0.2  OuterCtrl_Lvirt=0  InnerCtrl_K_p_V_cap_controller=0.17  InnerCtrl_K_i_V_cap_controller=4.24  InnerCtrl_K_p_I_conv_controller=0.5  InnerCtrl_K_i_I_conv_controller=2.5  InnerCtrl_v_conv_max=1.3  InnerCtrl_i_conv_max=1.32  InnerCtrl_Cff_V_cap_ctrl=disabled  InnerCtrl_Cff_I_conv_ctrl=disabled  InnerCtrl_K_ff_I_grid=enabled  InnerCtrl_K_ff_V_cap=enabled  InnerCtrl_i_lim_type=abc coordinate system  InnerCtrl_active_damping=enabled  InnerCtrl_AD_R_virt_pu=0.1
      settings: SourceProductName=tDMSquared
  Ground1 : Ground
  Ramp : simulink/Sources/Ramp  slope=400  start=0  InitialOutput=0
  Saturation : Saturate  UpperLimit=400
  Scope{14..19} (6 alike) : Scope
  Step1 : Step  Time=GFmAIC_Step_time  Before=GFmAIC_Initial_value  After=GFmAIC_Final_vlaue  SampleTime=GFmAIC_Sample_time
  a : PMIOPort  Side=Right
  b : PMIOPort  Port=2  Side=Right
  c : PMIOPort  Port=3  Side=Right
  wires:
  Bus Selector3/2 -> Scope15/1  "<Q_grid>"
  Bus Selector3/6 -> Scope19/1  "<I_grid_abc>"
  [AIC] -> Bus Selector3/1
  Bus Selector3/5 -> Scope18/1  "<V_grid_abc>"
  Grid_Forming_Converter_AIC/1 -> [AIC]
  Bus Selector3/3 -> Scope16/1  "<f>"
  Bus Selector3/4 -> Scope17/1  "<V_dc>"
  Bus Selector3/1 -> Scope14/1  "<P_grid>"
  Constant13/1 -> Grid_Forming_Converter_AIC/2
  Saturation/1 -> Grid_Forming_Converter_AIC/5
  Constant2/1 -> Grid_Forming_Converter_AIC/1
  Ramp/1 -> Saturation/1
  Constant12/1 -> Grid_Forming_Converter_AIC/4
  Ground1/1 -> Grid_Forming_Converter_AIC/6
  Constant14/1 -> Grid_Forming_Converter_AIC/3
  Step1/1 -> Grid_Forming_Converter_AIC/7
  connections:
  c/RConn1 -- Grid_Forming_Converter_AIC/RConn3
  a/RConn1 -- Grid_Forming_Converter_AIC/RConn1
  b/RConn1 -- Grid_Forming_Converter_AIC/RConn2

== system TEST_simulink/DER 1/SG ==
  Bus Selector2 : BusSelector  OutputSignals=electrical_SI.P_grid_SI,electrical_SI.Q_grid_SI,SG_SI.Frequency (Hz),electrical_SI.V_grid_SI
  Constant1 : Constant  Value=SG_P_primary
  Constant3 : Constant  Value=SG_f_set
  Constant5 : Constant  Value=SG_Q_set
  Constant7 : Constant  Value=SG_V_set_phph
  P_set_2 : Subsystem  Tag=STV Subsys  LoadFcn=sigbuilder_block('load');  StartFcn=sigbuilder_block('start');  StopFcn=sigbuilder_block('stop');  ClipboardFcn=sigbuilder_block('clipboard');  mask(Sigbuilder block){tuvar=[0:10]}
      mask help: Simulink:masks:SigbuilderBlock_MD
      mask init:
      | if ~strcmp(get_param(bdroot(gcbh),'SimulationStatus'),'stopped') tuvar = sigbuilder_block('maskInit'); end
      settings: CopyFcn=sigbuilder_block('copy');  DeleteFcn=sigbuilder_block('delete');  ModelCloseFcn=sigbuilder_block('modelClose');  PreSaveFcn=sigbuilder_block('preSave');  PauseFcn=sigbuilder_block('pause');  ContinueFcn=sigbuilder_block('continue');  NameChangeFcn=sigbuilder_block('namechange');  OpenFcn=sigbuilder_block('open',[747.75 145.5 551.25 360 ]);  CloseFcn=sigbuilder_block('close');
      mask Display: plot(0, 0, 100, 100,[2, 2, 32, 32, 2], [68, 8, 8, 68, 68],[32, 2], [38, 38], [32, 19, 2],[53, 60, 44], [32, 17, 17, 2],[16, 16, 31, 31]);txt = getActiveGroup(gcbh);text(2, 100, txt,'verticalAlignment', 'top');
  Scope{7..9,11} (4 alike) : Scope
  Step2 : Step  Time=SG_Step_time  Before=SG_Initial_value  After=SG_Final_vlaue  SampleTime=SG_Sample_time
  Synchronous_Generator : Model_DG_Synchronous_Generator/Synchronous_Generator  S_n=3.2e6  P_binst=2.0e6  V_n_phph=400  V_n_grid_phph=20e3  f_n=50  T_s_ctrl=1e-4  T_s_meas=1e-4  datatype='double'  SG_Reactances=[ 3.19 0.33 0.159 1.79 0.155 0.05 ]  SG_TimeConstants=[ 0.5 0.025 0.025 ]  SG_StatorResistance=0.00074  SG_mech=[ 0.366 0.01 2 ]  gov_type=IEEEG1 simplified  K_IEEEG1simp=10  T_IEEEG1simp=[ 0.2 0 0.1 0 ]  dP_maxmin_IEEEG1simp=[ 2 -2 ]  exciterModel=AC1A  QCtrl=Constant Voltage (no Q-Control)  K_p_QCtrl=0.5  K_i_QCtrl=0.4  uq0ref=1.0  qmax=0.33  umax=1.04  deadband=0  p_pu=[0.1, 0.5, 0.6, 0.9, 1.0]  q_pu=[0.0, 0.0, -0.05, -0.33, -0.33]  p1=[0.94, 0.33]  p2=[0.96, 0]  p3=[1.04, 0]  p4=[1.06, -0.33]  cosphi_ref=1  ind_cap_Q=Inductive behavior (capacitive Q infeed)  use_transformer=Grid coupling with transformer  RL_Trafo_GenSide=[ 0.002 0.08 ]  RL_Trafo_GridSide=[ 0.002 0.08 ]  Trafo_RmLm=[ 500 500 ]
      link override SG_Control/Exciter: LabelModeActiveChoice=AC1A
      link override SG_Control/Reactive_Power_Controller: LabelModeActiveChoice=const_V
      settings: SourceProductName=tDMSquared
  a : PMIOPort  Side=Right
  b : PMIOPort  Port=2  Side=Right
  c : PMIOPort  Port=3  Side=Right
  wires:
  Bus Selector2/4 -> Scope11/1  "<V_grid_SI>"
  Bus Selector2/2 -> Scope8/1  "<Q_grid_SI>"
  Bus Selector2/1 -> Scope7/1  "<P_grid_SI>"
  Bus Selector2/3 -> Scope9/1  "<Frequency (Hz)>"
  [sg] -> Bus Selector2/1
  Synchronous_Generator/1 -> [sg]
  Constant3/1 -> Synchronous_Generator/4
  Constant1/1 -> Synchronous_Generator/1
  P_set_2/1(P_set_2) -> Synchronous_Generator/2
  Constant5/1 -> Synchronous_Generator/3
  Constant7/1 -> Synchronous_Generator/5
  Step2/1 -> Synchronous_Generator/6
  connections:
  a/RConn1 -- Synchronous_Generator/RConn1
  c/RConn1 -- Synchronous_Generator/RConn3
  b/RConn1 -- Synchronous_Generator/RConn2
